simulink subsystem "valve"  (R2020a)
settings: Solver=VariableStepAuto  StartTime=0.0  StopTime=10.0  RelTol=1e-3
values from neighbouring files (symbols this model uses):
  dt = 0.01    [configure_simulation.m]    (also in test_kalman.m)
libraries: eePwmGenerator x1
settings Model: Creator=Philip  LastModifiedBy=Philip

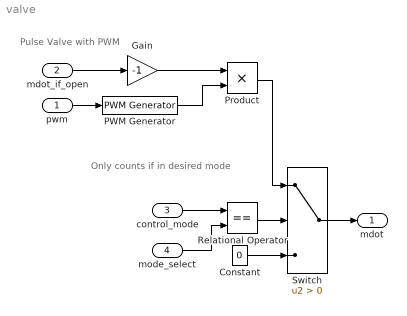
== system valve ==
  note: Pulse Valve with PWM
  note: Only counts if in desired mode
  pwm : Inport  OutDataTypeStr=double  PortDimensions=1
  mdot_if_open : Inport  Port=2  OutDataTypeStr=double  Unit=kg/s  PortDimensions=1
  control_mode : Inport  Port=3  OutDataTypeStr=Enum: enum_ControlMode
  mode_select : Inport  Port=4  OutDataTypeStr=Enum: enum_ControlMode
  Constant : Constant  Value=0
  Gain : Gain  Gain=-1
  PWM Generator : eePwmGenerator/PWM Generator  CarrCount=Up  Tper=pwm_period  Ts=dt
  Product : Product
  Relational Operator : RelationalOperator  Operator===  OutDataTypeStr=boolean  RndMeth=Simplest
  Switch : Switch  Criteria=u2 > Threshold
  mdot : Outport
  wires:
  Constant/1 -> Switch/3
  mdot_if_open/1 -> Gain/1
  pwm/1 -> PWM Generator/1
  Switch/1 -> mdot/1
  control_mode/1 -> Relational Operator/1
  mode_select/1 -> Relational Operator/2
  PWM Generator/1 -> Product/2
  Gain/1 -> Product/1
  Product/1 -> Switch/1
  Relational Operator/1 -> Switch/2
